simulink model "lab6_2"  (R2018b)
settings: Solver=VariableStepAuto  StartTime=0.0  StopTime=10.0  RelTol=1e-3
libraries: hdlsllib x1
settings Model: Creator=mllax8  LastModifiedBy=mllax8

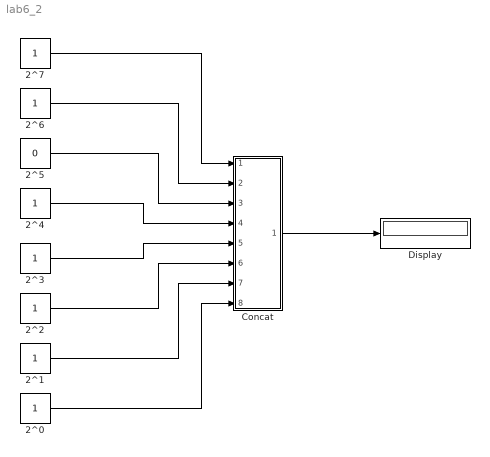
== system lab6_2 ==
  2^{0..4,6} (6 alike) : Constant  OutDataTypeStr=boolean
  2^5 : Constant  Value=0  OutDataTypeStr=boolean
  "2^7 " : Constant  OutDataTypeStr=boolean
  Concat : Subsystem
  Display : Display
      settings: Format=decimal (Stored Integer)
  wires:
  "2^7 "/1 -> Concat/1(2^7)
  2^6/1 -> Concat/2(2^6)
  2^5/1 -> Concat/3(2^5)
  2^4/1 -> Concat/4(2^4)
  2^3/1 -> Concat/5(2^3)
  2^2/1 -> Concat/6(2^2)
  2^1/1 -> Concat/7(2^1)
  2^0/1 -> Concat/8(2^0)
  Concat/1(unsign Int) -> Display/1

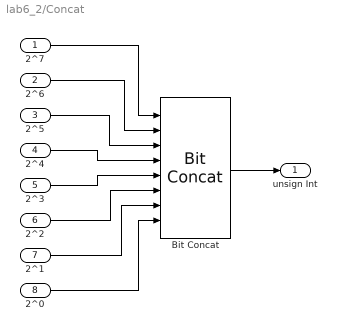
== system lab6_2/Concat ==
  2^7 : Inport
  2^6 : Inport  Port=2
  2^5 : Inport  Port=3
  2^4 : Inport  Port=4
  2^3 : Inport  Port=5
  2^2 : Inport  Port=6
  2^1 : Inport  Port=7
  2^0 : Inport  Port=8
  Bit Concat : hdlsllib/Logic and Bit Operations/Bit Concat  numInputs=8
      settings: SourceProductName=HDL Coder  SourceProductBaseCode=HD
  unsign Int : Outport
  wires:
  Bit Concat/1 -> unsign Int/1
  2^3/1 -> Bit Concat/5
  2^5/1 -> Bit Concat/3
  2^4/1 -> Bit Concat/4
  2^0/1 -> Bit Concat/8
  2^7/1 -> Bit Concat/1
  2^1/1 -> Bit Concat/7
  2^6/1 -> Bit Concat/2
  2^2/1 -> Bit Concat/6
